simulink model "S2_1"  (R2024b)
settings: Solver=FixedStepDiscrete  StartTime=0.0  StopTime=1  FixedStep=1e-5  RelTol=1e-3
libraries: simulink x1
settings Model: Creator=86195  LastModifiedBy=86195

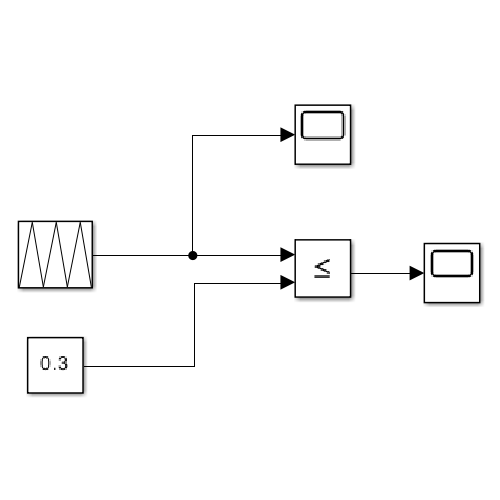
[thumbnail: Simulink's stored preview of the top-level diagram]
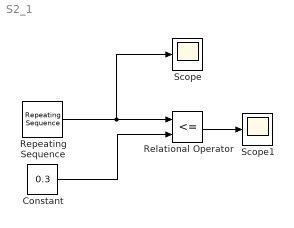
== system S2_1 ==
  Constant : Constant  Value=0.3
  Relational Operator : RelationalOperator  Operator=<=  OutDataTypeStr=boolean  RndMeth=Simplest  InputSameDT=off
  Repeating Sequence : simulink/Sources/Repeating Sequence  rep_seq_t=[0 1e-4 2e-4]  rep_seq_y=[0 1 0]
  Scope : Scope
  Scope1 : Scope
  wires:
  Repeating Sequence/1 -> Scope/1, Relational Operator/1
  Constant/1 -> Relational Operator/2
  Relational Operator/1 -> Scope1/1
